simulink model "Battery_Simulator"  (R2014a)
settings: Solver=FixedStepDiscrete  StartTime=0.0  StopTime=10.0  RelTol=1e-3
PreLoadFcn:
  | try, eval([bdroot '_setup']); catch, eval('model_setup', ''); end
InitFcn:
  | try, eval([bdroot '_setup']); catch, eval('model_setup', ''); end
undefined symbols (not defined in the file or in its folder): ECU565, motohawk_build_version, motohawk_trunc_name, motohawk_vardec_path
undefined symbols (not defined in the file): motohawk_get_target_image, motohawk_target_type
libraries: MotoHawk_lib x42, motohawk_annotations_lib x36
(part 1 of 2)
CloseFcn:
  | try, eval([bdroot '_close']); catch, eval('model_close', ''); end
Description:
  | Battery_Simulator
settings Model: MotoHawkBuildVersion=000  MotoHawkBuildStats=struct('TotalFLASH',{0},'TotalEEPROM',{0},'TotalRAM',{0},'AppFLASH',{0},'AppEEPROM',{0},'AppRAM',{0},'HeapRAM',{0},'BuildSuccessCount',{0},'BuildErrorCount',{0})  MotoHawkModelSavedName=Battery_Simulator  MotoHawkModelGUID=A0987AB7-E185-4605-B89A-B215F82E656D  MotoHawkModelOpenTime=2016 9 1 13 11 10.754  MotoHawkModelElapsedTime=6085.987  MotoHawkBuildInfo=struct('model_name',{'motohawk_template_model'},'motohawk_version',{'0.8.4_beta1'},'motohawk_component_version',{'0.0.3'},'matlab_version',{'6.5.1'},'build_version',{'000'},'layout_type',{'DEV'},'eri_table0_rev',{9},'max_eri_table_size',{255},'fptype',{0},'fgnd_base_period_ms',{5},'bgnd_base_period_ms',{50},'module_type',{'ECU555-80'},'processor_family',{'PPC'},'processor_type',{'MPC555'},'toolchain',{'GHS3.6'},'component',{0},'resource_file',{'PCM555Resources.h'},'archive_file',{'PCM.a'},'enable_build',{1},'flash_size',{458752},'ee_size',{8192},'ram_size',{26624},'decram_size',{0},'module_memory_def',{'MPC555_ModMemoryDef_Dev'},'use_debug_vardecs',{1},'root_build_dir',{'C:\MotoTron\MOTOHA~3\Blocks\Project'},'build_dir',{'C:\MotoTron\MOTOHA~3\Blocks\Project\motohawk_template_model_Build'},'dll_name',{'motohawk__000'},'srz_name',{'motohawk_template_model_000'},'fgnd_stack_size',{3072},'fgnd_angle_stack_size',{0},'bgnd_stack_size',{2048},'idle_stack_size',{1024},'irq_stack_size',{1536},'heap_size',{4096},'install_dll_dir',{'C:\ECUFiles\TDBDLL\'},'install_srz_dir',{'C:\ECUFiles\Programs\'},'motodevelopment_dir',{'C:\PROGRA~1\MotoTron\DEVELO~1\'},'motohawk_dir',{'C:\MotoTron\MOTOHA~3'},'ghs_dir',{'C:\GHS\ppc36'},'cw_dir',{'C:\Program Files\Freescale\CW for HC12 V4.5'},'matlab_root',{'C:\MATLAB6p5p1'},'model_guid',{'a528c725-4135-4734-9f-2c-07-29-37-5b-38'},'build_guid',{[]},'token_guid',{'6198A7A8FF044D4685C525ADFA06DAD5'})  Creator=cspenc  LastModifiedBy=ab9547
settings ConfigSet: Description="This Simulink Configuration Set is preconfigured  for the MotoHawk target \"ECU565-128\"."
settings OptimizationCC: InlineParams=on  InlineInvariantSignals=on  EnhancedBackFolding=on  ExpressionDepthLimit=2147483647  InitFltsAndDblsToZero=on  NoFixptDivByZeroProtection=on  EfficientFloat2IntCast=on  OptimizeModelRefInitCode=on  LifeSpan=1
settings DebuggingCC: UnderspecifiedInitializationDetection=Classic  SolverPrmCheckMsg=none  InheritedTsInSrcMsg=none  TasksWithSamePriorityMsg=none  FcnCallInpInsideContextMsg=EnableAllAsWarning  StateNameClashWarn=warning
settings HardwareCC: ProdLargestAtomicInteger=Integer  ProdLargestAtomicFloat=Float  ProdEndianess=BigEndian  ProdHWDeviceType=Specified
settings ModelReferenceCC: UpdateModelReferenceTargets=AssumeUpToDate  CheckModelReferenceTargetMessage=none  ModelReferenceNumInstancesAllowed=Zero
settings RTWCC: SystemTargetFile=motohawk_ert_rtw.tlc  MakeCommand=motohawk_make_rtw  TemplateMakefile=motohawk_ert_rtw.tmf  Description=MotoHawk(tm) Rapid Prototyping  ProcessScript=motohawk_ert_rtw_make_rtw_hook
settings CodeAppCC: IgnoreCustomStorageClasses=off  MaxIdLength=100  CustomSymbolStrType=$N$R$M  CustomSymbolStrField=$H$N$M  InternalIdentifier=Classic
settings STFCustomTargetCC: ERTMultiwordTypeDef=User defined  ERTMultiwordLength=0  ModelReferenceCompliant=off  ConcurrentExecutionCompliant=off  IncludeMdlTerminateFcn=off  CombineOutputUpdateFcns=on  SuppressErrorStatus=on  ERTCustomFileBanners=on  SupportContinuousTime=off  SupportNonInlinedSFcns=off  MATLABClassNameForMDSCustomization=Simulink.SoftwareTarget.ERTCustomization  GRTInterface=off  SystemTargetFile=motohawk_ert_rtw.tlc
settings ERTTargetCC: ERTMultiwordTypeDef=User defined  ERTMultiwordLength=0  GenerateSampleERTMain=off  ModelReferenceCompliant=off  IncludeMdlTerminateFcn=off  GeneratePreprocessorConditionals=Disable all  SuppressErrorStatus=on  ERTCustomFileTemplate=example_file_process.tlc

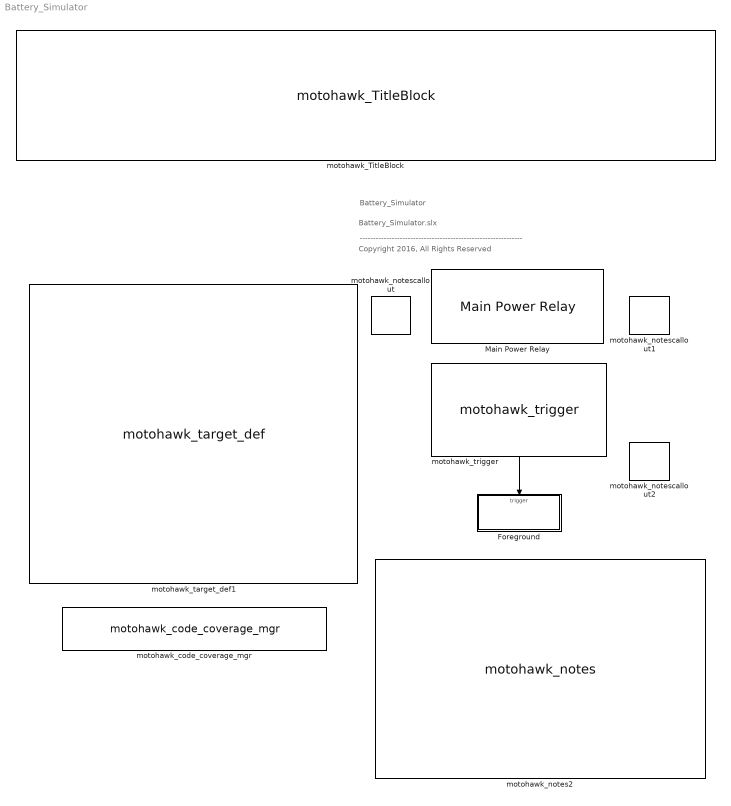
== system Battery_Simulator ==
  note: Battery_Simulator
  note: Battery_Simulator.slx
  note: -------------------------------------------------------------
  note: Copyright 2016, All Rights Reserved
  Foreground : Subsystem  TreatAsAtomicUnit=on
      mask init:
      | SampleTime = 0.005;
      | lbl = sprintf('%d ms', SampleTime * 1000);
      settings: RTWSystemCode=Nonreusable function  RTWFcnNameOpts=Use subsystem name  RTWFileNameOpts=Use function name
      mask Display: disp(lbl);
  Main Power Relay : MotoHawk_lib/Extra Development Blocks/Main Power Relay  on_delay_count=2  off_delay_count=5  ecup_threshold=100  group='System | Main Power Relay'
  motohawk_TitleBlock : motohawk_annotations_lib/motohawk_TitleBlock  BlockType_='Mototron_Title_Block'  ttl="[        strrep(get_param(bdroot, 'Description') , '_', '\\_')  '\\newline\\rm'        'Top-level root of model:  '   strrep(bdroot, '_', '\\_') '.mdl'        ]"  copyright="'THE INFORMATION CONTAINED IN THIS\\newlineDRAWING IS THE SOLE PROPERTY OF\\newlineWOODWARD.  ANY REPRODUCTION IN\\newline PART OR AS A WHOLE WITHOUT THE\\newlineWRITTEN PERMISSION OF WOODWARD\\newline IS PROHIBITED.\\fontsize{16}\\rm\\copyright\\rm\\fontsize{10} 2009'"  address='\fontsize{22}\it\fontname{Arial Black}Woodward \fontname{Arial}\fontsize{10}\newline1000 East Drake Road, Fort Collins, CO, 80525\newlinemcs.woodward.com (866) 588-0494'  image_file='mh.jpg'  pretty_print=on  edit_text="[strrep(get_param(bdroot, 'Description') , '_', '\\_')  '\\newline\\rm''Top-level root of model:  '   strrep(bdroot, '_', '\\_') '.mdl']"  edit_as=5
  motohawk_code_coverage_mgr : MotoHawk_lib/Extra Development Blocks/motohawk_code_coverage_mgr  codegen=Always Generate Code Coverage Code  group='System | Code Coverage'
  motohawk_notes2 : motohawk_annotations_lib/motohawk_notes  BlockType_='Mototron_Notes'  desc="'\\fontname{wingdings 2}u\\fontname{arial}  The existence of a Target Definition block\\newlinesomewhere in the model sets it up as a\\newlineMotoHawk project, capable of being built to a\\newlineMotoHawk capable target module.\\newline\\newline\\fontname{wingdings 2}v\\fontname{arial}  The Main Power Relay block monitors the\\newlinemodule power and controls the Main Power Relay\\newlineIt also performs startup and shutdown procedures\\newlinenecessary for EEPROM storage.  Most designs\\newlineshould contain this block\\newline\\newline\\fontname{wingdings 2}w\\fontname{arial}  All actions must be performed inside of a\\newlinefunction-call subsystem, triggered by a MotoHawk\\newlineentry-point trigger block, in order to be included in the\\newlinegenerated code.'"  edit_text="\\fontname{wingdings 2}u\\fontname{arial}  The existence of a Target Definition blocksomewhere in the model sets it up as aMotoHawk project, capable of being built to aMotoHawk capable target module.\\fontname{wingdings 2}v\\fontname{arial}  The Main Power Relay block monitors themodule power and controls the Main Power RelayIt also performs startup and shutdown proceduresnecessary for EEPROM storage.  Most designsshould contain this block\\fontname{wingdings 2}w\\fontname{arial}  All actions must be performed inside of afunction-call subsystem, triggered by a MotoHawkentry-point trigger block, in order to be included in thegenerated code."  edit_as=2
  motohawk_notescallout : motohawk_annotations_lib/motohawk_notescallout  BlockType_='Mototron_NoteCall'  desc='\bf1'
  motohawk_notescallout1 : motohawk_annotations_lib/motohawk_notescallout  BlockType_='Mototron_NoteCall'  desc='\bf2'
  motohawk_notescallout2 : motohawk_annotations_lib/motohawk_notescallout  BlockType_='Mototron_NoteCall'  desc='\bf3'
  motohawk_target_def1 : MotoHawk_lib/motohawk_target_def  Priority=-65535  target=ECU565-128  layout=DEV  fptype=single (32 bits)  fgnd_stack_size=3*1024  fgnd_angle_stack_size=0  bgnd_stack_size=2*1024  idle_stack_size=1024  irq_stack_size=1536  app_int_stack_size=1024  shutdown_stack_size=1024  heap_size=4*1024  show_margins=off  fgnd_stack_margin=(3*1024) * 0.1  fgnd_angle_stack_margin=0  bgnd_stack_margin=(2*1024) * 0.1  idle_stack_margin=(1024) * 0.1  irq_stack_margin=(1536) * 0.1  app_int_stack_margin=(1024) * 0.1  shutdown_stack_margin=(1024) * 0.1  heap_margin=(4*1024) * 0.1  comp_name=bdroot  comp_img='KVASER_CAN_USB.jpg'  comp_security=No Encryption  comp_build_pass='mhbuild'  comp_sim_pass='mhsim'  comp_multi=off  show_filenames=off  dll_name=motohawk_trunc_name(bdroot, ['_' motohawk_build_version], 50)  srz_name=motohawk_trunc_name(bdroot, ['_' motohawk_build_version], 50)  build_dir='.'  comp_dir='.'
  motohawk_trigger : MotoHawk_lib/Trigger Blocks/motohawk_trigger  Tag=Trigger  Priority=0  trig_name=[]  trigger=FGND_RTI_PERIODIC  priority_order=0  inherited=off  run_disabled=off  override_app_monitor=off  target=ECU565_128
  wires:
  motohawk_trigger/1 -> Foreground/Trigger

== system Battery_Simulator/Foreground ==
  f : TriggerPort  TriggerType=function-call
  Controller : Subsystem  mask(Display Image File){image_file=motohawk_get_target_image(motohawk_target_type(bdroot))}
      mask prompts: image_file "Image File"
      mask help:
      | Enter an image file on the current MATLAB path to display on this block.
      |
      | Double-clicking this block opens the contents of the subsystem.  Right-click and select 'Mask parameters...' to select a new image file.
      |
      | To use just the mask of this block in a model, but supply your own contents, break the link to the library.
      mask init:
      | try,
      | 	img = imread(image_file);
      | 	motohawk_block_image(gcb, image_file);
      | catch,
      | 	img = imread('image_not_found.jpg');
      | end
      settings: OpenFcn=open_system(gcb,'force')  MoveFcn=motohawk_block_image(gcb, motohawk_get_param_ws(gcb, 'image_file'));
      mask Display: image(img);
  Plant : Subsystem  mask(Display Image File){image_file='engine.jpg'}
      mask prompts: image_file "Image File"
      mask help:
      | Enter an image file on the current MATLAB path to display on this block.
      |
      | Double-clicking this block opens the contents of the subsystem.  Right-click and select 'Mask parameters...' to select a new image file.
      |
      | To use just the mask of this block in a model, but supply your own contents, break the link to the library.
      mask init:
      | try,
      | 	img = imread(image_file);
      | 	motohawk_block_image(gcb, image_file);
      | catch,
      | 	img = imread('image_not_found.jpg');
      | end
      settings: OpenFcn=open_system(gcb,'force')  MoveFcn=motohawk_block_image(gcb, motohawk_get_param_ws(gcb, 'image_file'));
      mask Display: image(img);
  motohawk_TitleBlock : motohawk_annotations_lib/motohawk_TitleBlock  BlockType_='Mototron_Title_Block'  ttl=[strrep(get_param(bdroot, 'Description') , '_', '\_') '\newline\rm' get_param(gcs, 'Name')]  copyright="'THE INFORMATION CONTAINED IN THIS\\newlineDRAWING IS THE SOLE PROPERTY OF\\newlineWOODWARD.  ANY REPRODUCTION IN\\newline PART OR AS A WHOLE WITHOUT THE\\newlineWRITTEN PERMISSION OF WOODWARD\\newline IS PROHIBITED.\\fontsize{16}\\rm\\copyright\\rm\\fontsize{10} 2009'"  address='\fontsize{22}\it\fontname{Arial Black}Woodward \fontname{Arial}\fontsize{10}\newline1000 East Drake Road, Fort Collins, CO, 80525\newlinemcs.woodward.com (866) 588-0494'  image_file='mh.jpg'  pretty_print=on  edit_text=[strrep(get_param(bdroot, 'Description') , '_', '\_') '\newline\rm' get_param(gcs, 'Name')]  edit_as=5
  motohawk_code_coverage : MotoHawk_lib/Extra Development Blocks/motohawk_code_coverage
  wires:
  Plant/1(SensorBus) -> Controller/1(Sensors)
  Controller/1(Actuators) -> Plant/1(ActuatorBus)

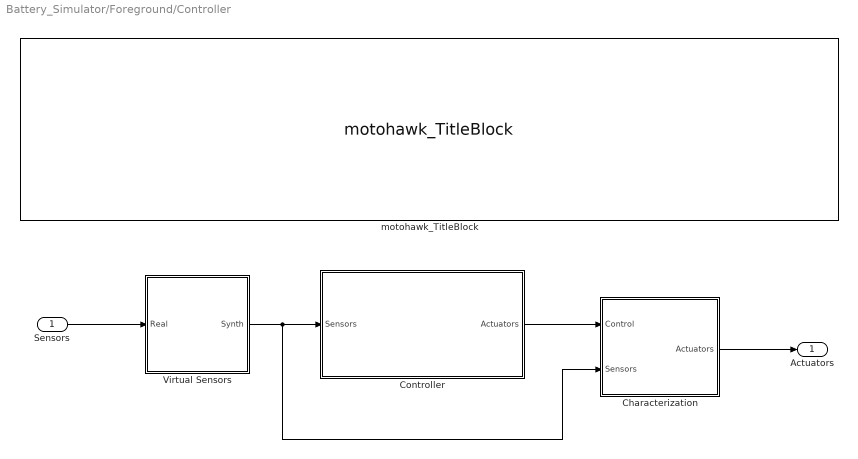
== system Battery_Simulator/Foreground/Controller ==
  Sensors : Inport
  Characterization : Subsystem
  Controller : Subsystem
  Virtual Sensors : Subsystem
  motohawk_TitleBlock : motohawk_annotations_lib/motohawk_TitleBlock  BlockType_='Mototron_Title_Block'  ttl=[get_param(bdroot, 'Description') '\rm\newlineTop-level design of Controller\newlineVirtual Sensors model signals that are not available as H/W sensors\newlineCharacterization converts or linearizes Controller units to actuator units\newline']  copyright="'THE INFORMATION CONTAINED IN THIS\\newlineDRAWING IS THE SOLE PROPERTY OF\\newlineWOODWARD.  ANY REPRODUCTION IN\\newline PART OR AS A WHOLE WITHOUT THE\\newlineWRITTEN PERMISSION OF WOODWARD\\newline IS PROHIBITED.\\fontsize{16}\\rm\\copyright\\rm\\fontsize{10} 2009'"  address='\fontsize{22}\it\fontname{Arial Black}Woodward \fontname{Arial}\fontsize{10}\newline1000 East Drake Road, Fort Collins, CO, 80525\newlinemcs.woodward.com (866) 588-0494'  image_file='mh.jpg'  pretty_print=on  edit_text=|  edit_as=6
      | [get_param(bdroot, 'Description') '\rm
      | 
      | 
      | Top-level design of Controller
      | 
      | 
      | Virtual Sensors model signals that are not available as H/W sensors
      | 
      | 
      | Characterization converts or linearizes Controller units to actuator units
      | 
      | 
      | ']
  Actuators : Outport
  wires:
  Controller/1(Actuators) -> Characterization/1(Control)
  Virtual Sensors/1(Synth) -> Controller/1(Sensors), Characterization/2(Sensors)
  Sensors/1 -> Virtual Sensors/1(Real)
  Characterization/1(Actuators) -> Actuators/1

== system Battery_Simulator/Foreground/Plant ==
  ActuatorBus : Inport
  Actuators : Subsystem
  Sensors : Subsystem
  motohawk_TitleBlock : motohawk_annotations_lib/motohawk_TitleBlock  BlockType_='Mototron_Title_Block'  ttl=[get_param(bdroot, 'Description') '\rm\newlineRead H/W sensors and Drive H/W actuators\newlineThe Sensors and Actuators busses should contain signals in engineering units\newline']  copyright="'THE INFORMATION CONTAINED IN THIS\\newlineDRAWING IS THE SOLE PROPERTY OF\\newlineWOODWARD.  ANY REPRODUCTION IN\\newline PART OR AS A WHOLE WITHOUT THE\\newlineWRITTEN PERMISSION OF WOODWARD\\newline IS PROHIBITED.\\fontsize{16}\\rm\\copyright\\rm\\fontsize{10} 2009'"  address='\fontsize{22}\it\fontname{Arial Black}Woodward \fontname{Arial}\fontsize{10}\newline1000 East Drake Road, Fort Collins, CO, 80525\newlinemcs.woodward.com (866) 588-0494'  image_file='mh.jpg'  pretty_print=on  edit_text=|  edit_as=6
      | [get_param(bdroot, 'Description') '\rm
      | 
      | 
      | Read H/W sensors and Drive H/W actuators
      | 
      | 
      | The Sensors and Actuators busses should contain signals in engineering units
      | 
      | 
      | ']
  SensorBus : Outport
  wires:
  Sensors/1(Sensors) -> SensorBus/1
  ActuatorBus/1 -> Actuators/1(Actuators)

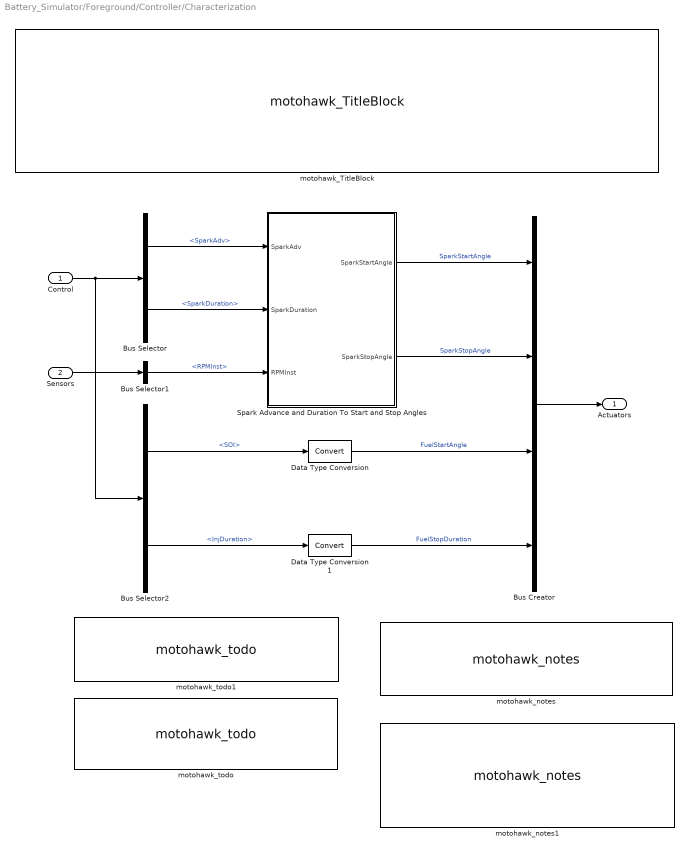
== system Battery_Simulator/Foreground/Controller/Characterization ==
  Control : Inport
  Sensors : Inport  Port=2
  Bus Creator : BusCreator
  Bus Selector : BusSelector  OutputSignals=SparkAdv,SparkDuration
  Bus Selector1 : BusSelector  OutputSignals=RPMInst
  Bus Selector2 : BusSelector  OutputSignals=SOI,InjDuration
  Data Type Conversion : DataTypeConversion  SaturateOnIntegerOverflow=on  RndMeth=Zero
  Data Type Conversion1 : DataTypeConversion  SaturateOnIntegerOverflow=on  RndMeth=Zero
  Spark Advance and Duration To Start and Stop Angles : Subsystem
  motohawk_TitleBlock : motohawk_annotations_lib/motohawk_TitleBlock  BlockType_='Mototron_Title_Block'  ttl=[get_param(bdroot, 'Description') '\rm\newlineActuator Characterization\newlineConverts or linearizes controller units to actuator units\newline']  copyright="'THE INFORMATION CONTAINED IN THIS\\newlineDRAWING IS THE SOLE PROPERTY OF\\newlineWOODWARD.  ANY REPRODUCTION IN\\newline PART OR AS A WHOLE WITHOUT THE\\newlineWRITTEN PERMISSION OF WOODWARD\\newline IS PROHIBITED.\\fontsize{16}\\rm\\copyright\\rm\\fontsize{10} 2009'"  address='\fontsize{22}\it\fontname{Arial Black}Woodward \fontname{Arial}\fontsize{10}\newline1000 East Drake Road, Fort Collins, CO, 80525\newlinemcs.woodward.com (866) 588-0494'  image_file='mh.jpg'  pretty_print=on  edit_text=|  edit_as=6
      | [get_param(bdroot, 'Description') '\rm
      | 
      | 
      | Actuator Characterization
      | 
      | 
      | Converts or linearizes controller units to actuator units
      | 
      | 
      | ']
  motohawk_notes : motohawk_annotations_lib/motohawk_notes  BlockType_='Mototron_Notes'  desc='- Outputs from here are still entirely in engineering\newlineunits, but are converted from a form used by the\newlinecontroller to one required by the physical actuators'  edit_text=|  edit_as=0
      | - Outputs from here are still entirely in engineering
      | 
      | 
      | units, but are converted from a form used by the
      | 
      | 
      | controller to one required by the physical actuators
  motohawk_notes1 : motohawk_annotations_lib/motohawk_notes  BlockType_='Mototron_Notes'  desc='- This is a good place to put a PID controller that\newlineis always enabled, such as an electronic throttle\newlinecontroller (ETC)\newline\newline- The controller outputs a desired setpoint,\newlinea block in this subsystem performs the\newlineclosed-loop control to that position.'  edit_text=|  edit_as=0
      | - This is a good place to put a PID controller that
      | 
      | 
      | is always enabled, such as an electronic throttle
      | 
      | 
      | controller (ETC)
      | 
      | 
      | 
      | 
      | 
      | - The controller outputs a desired setpoint,
      | 
      | 
      | a block in this subsystem performs the
      | 
      | 
      | closed-loop control to that position.
  motohawk_todo : motohawk_annotations_lib/motohawk_todo  BlockType_='Mototron_ToDo'  desc='\fontsize{16}\bfTo Do:\newlineConvert from desired controller units\newlineto those required by each actuator.'  edit_text=|  edit_as=2
      | \fontsize{16}\bfTo Do:
      | 
      | 
      | Convert from desired controller units
      | 
      | 
      | to those required by each actuator.
  motohawk_todo1 : motohawk_annotations_lib/motohawk_todo  BlockType_='Mototron_ToDo'  desc='\fontsize{16}\bfTo Do:\newlinePass-through actuators\newlinethat do not require modification.'  edit_text=|  edit_as=2
      | \fontsize{16}\bfTo Do:
      | 
      | 
      | Pass-through actuators
      | 
      | 
      | that do not require modification.
  Actuators : Outport
  wires:
  Spark Advance and Duration To Start and Stop Angles/1(SparkStartAngle) -> Bus Creator/1  "SparkStartAngle"
  Bus Creator/1 -> Actuators/1
  Spark Advance and Duration To Start and Stop Angles/2(SparkStopAngle) -> Bus Creator/2  "SparkStopAngle"
  Bus Selector2/1 -> Data Type Conversion/1  "<SOI>"
  Bus Selector2/2 -> Data Type Conversion1/1  "<InjDuration>"
  Sensors/1 -> Bus Selector1/1
  Bus Selector1/1 -> Spark Advance and Duration To Start and Stop Angles/3(RPMInst)  "<RPMInst>"
  Bus Selector/1 -> Spark Advance and Duration To Start and Stop Angles/1(SparkAdv)  "<SparkAdv>"
  Bus Selector/2 -> Spark Advance and Duration To Start and Stop Angles/2(SparkDuration)  "<SparkDuration>"
  Control/1 -> Bus Selector/1, Bus Selector2/1
  Data Type Conversion/1 -> Bus Creator/3  "FuelStartAngle"
  Data Type Conversion1/1 -> Bus Creator/4  "FuelStopDuration"

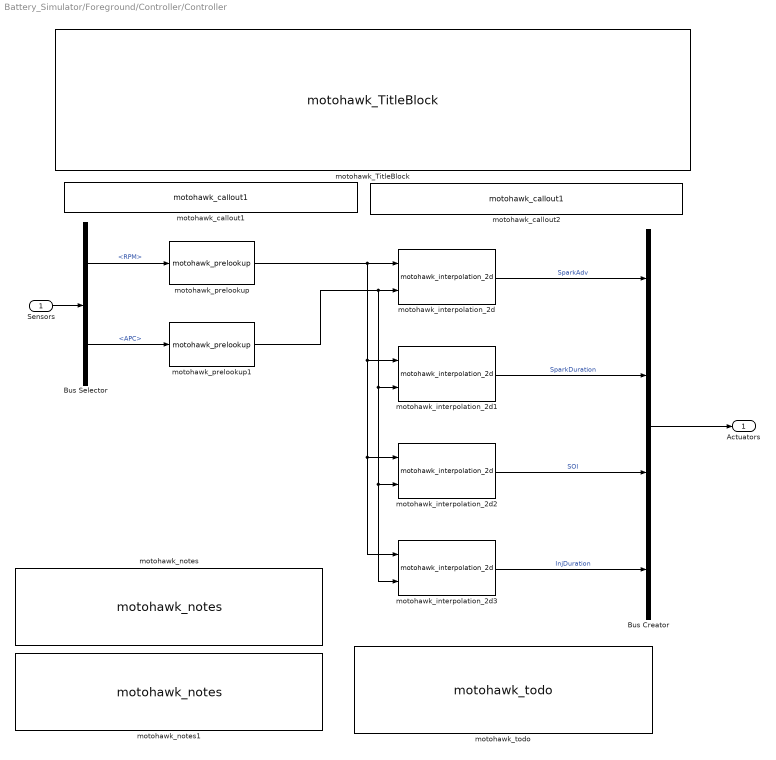
== system Battery_Simulator/Foreground/Controller/Controller ==
  Sensors : Inport
  Bus Creator : BusCreator
  Bus Selector : BusSelector  OutputSignals=RPM,APC
  motohawk_TitleBlock : motohawk_annotations_lib/motohawk_TitleBlock  BlockType_='Mototron_Title_Block'  ttl=[get_param(bdroot, 'Description') '\rm\newlineEngine control system\newlineConsists of simple tables for spark and fuel\newline']  copyright="'THE INFORMATION CONTAINED IN THIS\\newlineDRAWING IS THE SOLE PROPERTY OF\\newlineWOODWARD.  ANY REPRODUCTION IN\\newline PART OR AS A WHOLE WITHOUT THE\\newlineWRITTEN PERMISSION OF WOODWARD\\newline IS PROHIBITED.\\fontsize{16}\\rm\\copyright\\rm\\fontsize{10} 2009'"  address='\fontsize{22}\it\fontname{Arial Black}Woodward \fontname{Arial}\fontsize{10}\newline1000 East Drake Road, Fort Collins, CO, 80525\newlinemcs.woodward.com (866) 588-0494'  image_file='mh.jpg'  pretty_print=on  edit_text=|  edit_as=6
      | [get_param(bdroot, 'Description') '\rm
      | 
      | 
      | Engine control system
      | 
      | 
      | Consists of simple tables for spark and fuel
      | 
      | 
      | ']
  motohawk_callout1 : motohawk_annotations_lib/motohawk_callout1  BlockType_='Mototron_harea'  desc='Prelookups for each axis of the tables'  edit_text=Prelookups for each axis of the tables  edit_as=0
  motohawk_callout2 : motohawk_annotations_lib/motohawk_callout1  BlockType_='Mototron_harea'  desc='2-D interpolated tables for each actuator'  edit_text=2-D interpolated tables for each actuator  edit_as=0
  motohawk_interpolation_2d : MotoHawk_lib/Lookup Tables/motohawk_interpolation_2d  nam='SparkAdv'  table_data=zeros(11,11)  show_more=off  data_type=Inherit from 'Table Data'  storage=NonAdaptive  read_level=1  write_level=1  ovr_cals=on  use_help=off  help=''  units=''  use_min_max=off  min_val=-inf  max_val=inf  use_precision=off  precision=''  gain=1  offset=0  exp=1  use_links=off  row_prelookup_block=''  col_prelookup_block=''  output_name=''  use_mototune_group=off  mototune_group=motohawk_vardec_path(gcb)  data_stores=motohawk_sfun_interpolation_2d_data_stores
  motohawk_interpolation_2d1 : MotoHawk_lib/Lookup Tables/motohawk_interpolation_2d  nam='SparkDuration'  table_data=ones(11,11)  show_more=off  data_type=Inherit from 'Table Data'  storage=NonAdaptive  read_level=1  write_level=1  ovr_cals=on  use_help=off  help=''  units=''  use_min_max=off  min_val=-inf  max_val=inf  use_precision=off  precision=''  gain=1  offset=0  exp=1  use_links=off  row_prelookup_block=''  col_prelookup_block=''  output_name=''  use_mototune_group=off  mototune_group=motohawk_vardec_path(gcb)  data_stores=motohawk_sfun_interpolation_2d_data_stores
  motohawk_interpolation_2d2 : MotoHawk_lib/Lookup Tables/motohawk_interpolation_2d  nam='SOI'  table_data=zeros(11,11)  show_more=off  data_type=Inherit from 'Table Data'  storage=NonAdaptive  read_level=1  write_level=1  ovr_cals=on  use_help=off  help=''  units=''  use_min_max=off  min_val=-inf  max_val=inf  use_precision=off  precision=''  gain=1  offset=0  exp=1  use_links=off  row_prelookup_block=''  col_prelookup_block=''  output_name=''  use_mototune_group=off  mototune_group=motohawk_vardec_path(gcb)  data_stores=motohawk_sfun_interpolation_2d_data_stores
  motohawk_interpolation_2d3 : MotoHawk_lib/Lookup Tables/motohawk_interpolation_2d  nam='InjDuration'  table_data=5*ones(11,11)  show_more=off  data_type=Inherit from 'Table Data'  storage=NonAdaptive  read_level=1  write_level=1  ovr_cals=on  use_help=off  help=''  units=''  use_min_max=off  min_val=-inf  max_val=inf  use_precision=off  precision=''  gain=1  offset=0  exp=1  use_links=off  row_prelookup_block=''  col_prelookup_block=''  output_name=''  use_mototune_group=off  mototune_group=motohawk_vardec_path(gcb)  data_stores=motohawk_sfun_interpolation_2d_data_stores
  motohawk_notes : motohawk_annotations_lib/motohawk_notes  BlockType_='Mototron_Notes'  desc='Simplify as much as possible, by offloading work to the\newlineVirtual Sensors and Actuator Characterization subsystems'  edit_text=|  edit_as=0
      | Simplify as much as possible, by offloading work to the
      | 
      | 
      | Virtual Sensors and Actuator Characterization subsystems
  motohawk_notes1 : motohawk_annotations_lib/motohawk_notes  BlockType_='Mototron_Notes'  desc='If the controller contains multiple states,\newlinecreate a StateFlow representation of the state machine here.'  edit_text=|  edit_as=0
      | If the controller contains multiple states,
      | 
      | 
      | create a StateFlow representation of the state machine here.
  motohawk_prelookup : MotoHawk_lib/Lookup Tables/motohawk_prelookup  nam='RPM'  breakpoint_data=[0:500:5000]  show_more=on  data_type=Inherit from 'Table Data'  storage=Constant  read_level=1  write_level=1  ovr_cals=on  use_help=off  help=''  units=''  use_min_max=off  min_val=-inf  max_val=inf  use_precision=off  precision=''  gain=1  offset=0  exp=1  use_links=on  input_name='RPM'  use_mototune_group=off  mototune_group=motohawk_vardec_path(gcb)  data_stores=motohawk_sfun_prelookup_data_stores
  motohawk_prelookup1 : MotoHawk_lib/Lookup Tables/motohawk_prelookup  nam='APC'  breakpoint_data=[0:0.5:5]  show_more=on  data_type=Inherit from 'Table Data'  storage=Constant  read_level=1  write_level=1  ovr_cals=on  use_help=off  help=''  units=''  use_min_max=off  min_val=-inf  max_val=inf  use_precision=off  precision=''  gain=1  offset=0  exp=1  use_links=on  input_name='APC'  use_mototune_group=off  mototune_group=motohawk_vardec_path(gcb)  data_stores=motohawk_sfun_prelookup_data_stores
  motohawk_todo : motohawk_annotations_lib/motohawk_todo  BlockType_='Mototron_ToDo'  desc='\fontsize{16}\bfTo Do:\newlinePerform the actions required by the controller.'  edit_text=|  edit_as=2
      | \fontsize{16}\bfTo Do:
      | 
      | 
      | Perform the actions required by the controller.
  Actuators : Outport
  wires:
  Bus Creator/1 -> Actuators/1
  motohawk_interpolation_2d/1 -> Bus Creator/1  "SparkAdv"
  motohawk_interpolation_2d1/1 -> Bus Creator/2  "SparkDuration"
  motohawk_interpolation_2d2/1 -> Bus Creator/3  "SOI"
  motohawk_interpolation_2d3/1 -> Bus Creator/4  "InjDuration"
  Sensors/1 -> Bus Selector/1
  Bus Selector/1 -> motohawk_prelookup/1  "<RPM>"
  Bus Selector/2 -> motohawk_prelookup1/1  "<APC>"
  motohawk_prelookup/1 -> motohawk_interpolation_2d/1, motohawk_interpolation_2d1/1, motohawk_interpolation_2d2/1, motohawk_interpolation_2d3/1
  motohawk_prelookup1/1 -> motohawk_interpolation_2d/2, motohawk_interpolation_2d1/2, motohawk_interpolation_2d2/2, motohawk_interpolation_2d3/2

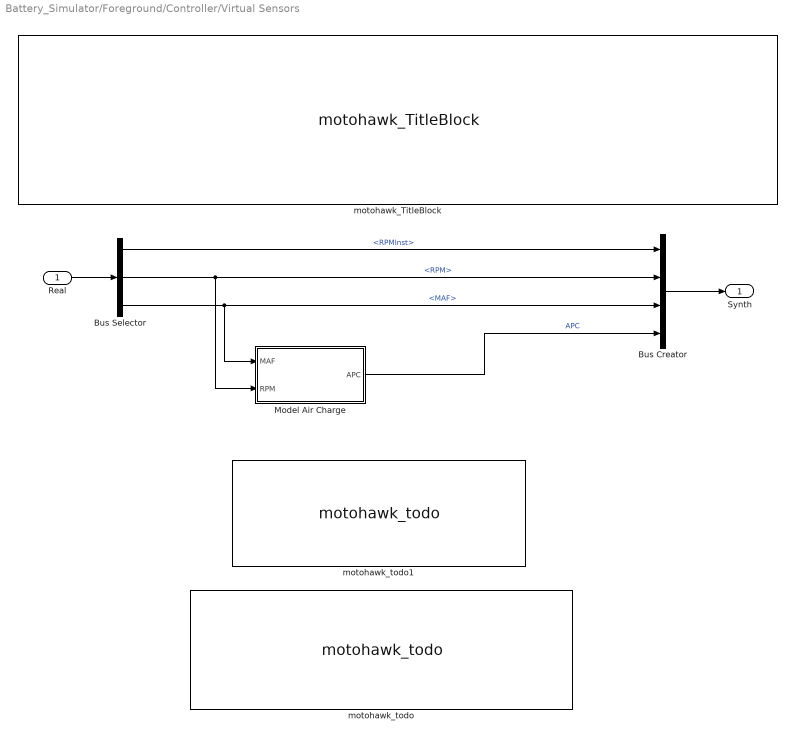
== system Battery_Simulator/Foreground/Controller/Virtual Sensors ==
  Real : Inport
  Bus Creator : BusCreator
  Bus Selector : BusSelector  OutputSignals=RPMInst,RPM,MAF
  Model Air Charge : Subsystem
  motohawk_TitleBlock : motohawk_annotations_lib/motohawk_TitleBlock  BlockType_='Mototron_Title_Block'  ttl=[get_param(bdroot, 'Description') '\newline\rmVirtual Sensors\newlineModel signals that are not available as H/W sensors,\newlinebut that would be used by the controller if they were physically available']  copyright="'THE INFORMATION CONTAINED IN THIS\\newlineDRAWING IS THE SOLE PROPERTY OF\\newlineWOODWARD.  ANY REPRODUCTION IN\\newline PART OR AS A WHOLE WITHOUT THE\\newlineWRITTEN PERMISSION OF WOODWARD\\newline IS PROHIBITED.\\fontsize{16}\\rm\\copyright\\rm\\fontsize{10} 2009'"  address='\fontsize{22}\it\fontname{Arial Black}Woodward \fontname{Arial}\fontsize{10}\newline1000 East Drake Road, Fort Collins, CO, 80525\newlinemcs.woodward.com (866) 588-0494'  image_file='mh.jpg'  pretty_print=on  edit_text="strrep([get_param(bdroot, 'Description')  '\\rm\\newline'  get_param(gcs, 'Name')], '_', '\\_')"  edit_as=255
  motohawk_todo : motohawk_annotations_lib/motohawk_todo  BlockType_='Mototron_ToDo'  desc="'\\fontsize{16}\\bfTo Do:\\newlineModel Extra \"Virtual\" Sensors\\newlineso that the downstream controller can\\newlineuse modeled variables as sensor values'"  edit_text=|  edit_as=2
      | \fontsize{16}\bfTo Do:
      | 
      | 
      | Model Extra "Virtual" Sensors
      | 
      | 
      | so that the downstream controller can
      | 
      | 
      | use modeled variables as sensor values
  motohawk_todo1 : motohawk_annotations_lib/motohawk_todo  BlockType_='Mototron_ToDo'  desc='\fontsize{16}\bfTo Do:\newlinePass-through sensors\newlinethat do not require modification.'  edit_text=|  edit_as=2
      | \fontsize{16}\bfTo Do:
      | 
      | 
      | Pass-through sensors
      | 
      | 
      | that do not require modification.
  Synth : Outport
  wires:
  Real/1 -> Bus Selector/1
  Bus Selector/1 -> Bus Creator/1  "<RPMInst>"
  Bus Selector/2 -> Bus Creator/2, Model Air Charge/2(RPM)  "<RPM>"
  Bus Selector/3 -> Bus Creator/3, Model Air Charge/1(MAF)  "<MAF>"
  Model Air Charge/1(APC) -> Bus Creator/4  "APC"
  Bus Creator/1 -> Synth/1

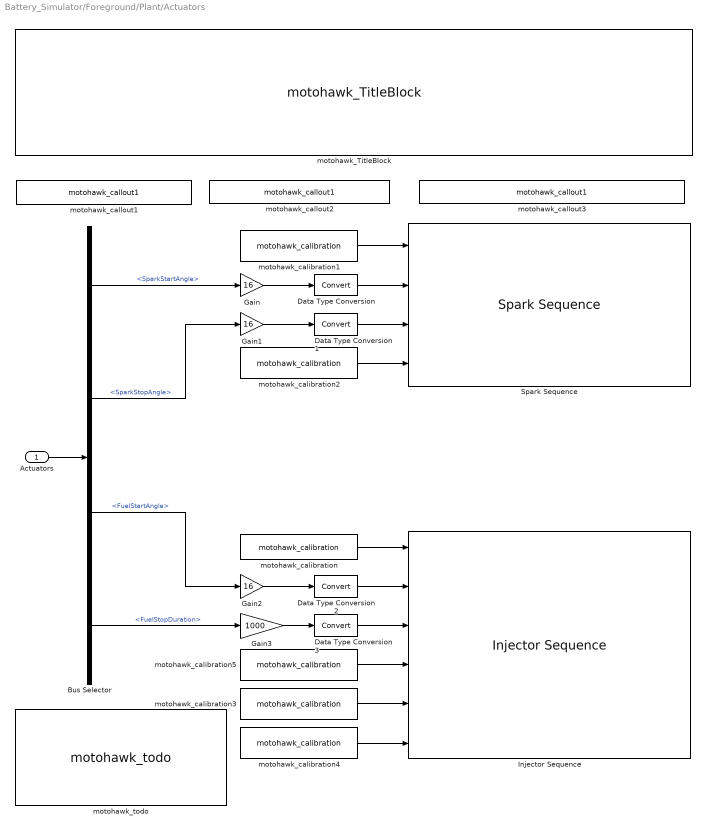
== system Battery_Simulator/Foreground/Plant/Actuators ==
  Actuators : Inport
  Bus Selector : BusSelector  OutputSignals=SparkStartAngle,SparkStopAngle,FuelStartAngle,FuelStopDuration
  Data Type Conversion{,1..3} (4 alike) : DataTypeConversion  SaturateOnIntegerOverflow=on  RndMeth=Zero
  Gain : Gain  Gain=16  SaturateOnIntegerOverflow=on  OutDataTypeStr=Inherit: Same as input  ParamDataTypeStr=Inherit: Same as input
  Gain1 : Gain  Gain=16  SaturateOnIntegerOverflow=on  OutDataTypeStr=Inherit: Same as input  ParamDataTypeStr=Inherit: Same as input
  Gain2 : Gain  Gain=16  SaturateOnIntegerOverflow=on  OutDataTypeStr=Inherit: Same as input  ParamDataTypeStr=Inherit: Same as input
  Gain3 : Gain  Gain=1000  SaturateOnIntegerOverflow=on  OutDataTypeStr=Inherit: Same as input  ParamDataTypeStr=Inherit: Same as input
  Injector Sequence : MotoHawk_lib/Advanced Digital I//O/Injector Sequence  text_resource=FINJ1  code_resource=NONE  val_resource=-1  target=ECU565-128  resource_enum_str=(None)=-1,FINJ1=12,FINJ2=13,FINJ3=14,FINJ4=15,FINJ5=16,FINJ6=17,FINJ7=18,FINJ8=19,FINJ9=20,FINJ10=21,FINJ11=22,FINJ12=23  sequence_type=Standard (Injector per cylinder)  behavior=Standard  update_mode=OS  granularity=Fine  use_makeup=off  min_eoi_soi_angle=90  use_diag=off  show_trans_enable=off  min_duration_mode=Static  min_duration=1.5  use_vardec=off  nam='INJ_'  read_level=1  write_level=1  group='System | I/O Pins | Injector Config'
  Spark Sequence : MotoHawk_lib/Advanced Digital I//O/Spark Sequence  text_resource=EST 1  code_resource=NONE  val_resource=-1  target=ECU565-128  resource_enum_str=(None)=-1,EST 1=36,EST 2=37,EST 3=38,EST 4=39,EST 5=40,EST 6=41,EST 7=42,EST 8=43,EST 9=44,EST 10=45,EST 11=46,EST 12=47,EST 13=48,EST 14=49,EST 15=50,EST 16=51  sequence_type=Standard (Coil per cylinder)  stop_mode=Angle Controlled  update_mode=OS  granularity=Fine  min_duration_mode=Static  min_duration=1.5  use_diag=off  open_threshold=500  use_vardec=off  nam='EST_'  read_level=1  write_level=1  group='System | I/O Pins | Spark Config'
  motohawk_TitleBlock : motohawk_annotations_lib/motohawk_TitleBlock  BlockType_='Mototron_Title_Block'  ttl=[get_param(bdroot, 'Description') '\rm\newlineSample H/W sensors, such as:\newlineA/D converters, digital inputs, frequency inputs, and engine encoder\newline']  copyright="'THE INFORMATION CONTAINED IN THIS\\newlineDRAWING IS THE SOLE PROPERTY OF\\newlineWOODWARD.  ANY REPRODUCTION IN\\newline PART OR AS A WHOLE WITHOUT THE\\newlineWRITTEN PERMISSION OF WOODWARD\\newline IS PROHIBITED.\\fontsize{16}\\rm\\copyright\\rm\\fontsize{10} 2009'"  address='\fontsize{22}\it\fontname{Arial Black}Woodward \fontname{Arial}\fontsize{10}\newline1000 East Drake Road, Fort Collins, CO, 80525\newlinemcs.woodward.com (866) 588-0494'  image_file='mh.jpg'  pretty_print=on  edit_text=|  edit_as=6
      | [get_param(bdroot, 'Description') '\rm
      | 
      | 
      | Sample H/W sensors, such as:
      | 
      | 
      | A/D converters, digital inputs, frequency inputs, and engine encoder
      | 
      | 
      | ']
  motohawk_calibration : MotoHawk_lib/Calibration & Probing Blocks/motohawk_calibration  nam='InjectorEnable'  val=false  storage=Display  show_more=on  name_source=Use Parameter  data_type=Inherit from 'Default Value'  read_level=1  write_level=1  ovr_cals=on  view_as=Enumeration  enum_struct={'Disabled', 'Enabled'}  vector_style=Wide Row  use_help_units=off  help=''  units=''  use_header_enum=off  row_header_enum={}  col_header_enum={}  use_min_max=off  min_val=-inf  max_val=inf  use_precision=off  precision=''  gain=1  offset=0  exp=1  use_mototune_group=off  mototune_group=motohawk_vardec_path(gcb)  data_stores=motohawk_sfun_calibration_data_stores
  motohawk_calibration1 : MotoHawk_lib/Calibration & Probing Blocks/motohawk_calibration  nam='SparkEnable'  val=false  storage=Display  show_more=on  name_source=Use Parameter  data_type=Inherit from 'Default Value'  read_level=1  write_level=1  ovr_cals=on  view_as=Enumeration  enum_struct={'Disabled', 'Enabled'}  vector_style=Wide Row  use_help_units=off  help=''  units=''  use_header_enum=off  row_header_enum={}  col_header_enum={}  use_min_max=off  min_val=-inf  max_val=inf  use_precision=off  precision=''  gain=1  offset=0  exp=1  use_mototune_group=off  mototune_group=motohawk_vardec_path(gcb)  data_stores=motohawk_sfun_calibration_data_stores
  motohawk_calibration2 : MotoHawk_lib/Calibration & Probing Blocks/motohawk_calibration  nam='SparkMaxDuration'  val=5000  storage=Calibration  show_more=on  name_source=Use Parameter  data_type=Inherit via back propagation  read_level=1  write_level=1  ovr_cals=on  view_as=Number  enum_struct={'Disabled', 'Enabled'}  vector_style=Wide Row  use_help_units=on  help="'Maximum duration for a spark pulse.  Must be a multiple of 5ms'"  units='us'  use_header_enum=off  row_header_enum={}  col_header_enum={}  use_min_max=off  min_val=-inf  max_val=inf  use_precision=off  precision=''  gain=1  offset=0  exp=1  use_mototune_group=off  mototune_group=motohawk_vardec_path(gcb)  data_stores=motohawk_sfun_calibration_data_stores
  motohawk_calibration3 : MotoHawk_lib/Calibration & Probing Blocks/motohawk_calibration  nam='InjectorMaxDuration'  val=500000  storage=Calibration  show_more=on  name_source=Use Parameter  data_type=Inherit via back propagation  read_level=1  write_level=1  ovr_cals=on  view_as=Number  enum_struct={'Disabled', 'Enabled'}  vector_style=Wide Row  use_help_units=on  help="'Maximum duration for an injector pulse.  Must be a multiple of 5ms'"  units='us'  use_header_enum=off  row_header_enum={}  col_header_enum={}  use_min_max=off  min_val=-inf  max_val=inf  use_precision=off  precision=''  gain=1  offset=0  exp=1  use_mototune_group=off  mototune_group=motohawk_vardec_path(gcb)  data_stores=motohawk_sfun_calibration_data_stores
  motohawk_calibration4 : MotoHawk_lib/Calibration & Probing Blocks/motohawk_calibration  nam='InjectorElectricalOffset'  val=0  storage=Calibration  show_more=on  name_source=Use Parameter  data_type=Inherit via back propagation  read_level=1  write_level=1  ovr_cals=on  view_as=Number  enum_struct={'Disabled', 'Enabled'}  vector_style=Wide Row  use_help_units=on  help='Extra duration added to each generated pulse to account for the injector turn on and turn off time'  units='us'  use_header_enum=off  row_header_enum={}  col_header_enum={}  use_min_max=off  min_val=-inf  max_val=inf  use_precision=off  precision=''  gain=1  offset=0  exp=1  use_mototune_group=off  mototune_group=motohawk_vardec_path(gcb)  data_stores=motohawk_sfun_calibration_data_stores
  motohawk_calibration5 : MotoHawk_lib/Calibration & Probing Blocks/motohawk_calibration  nam='InjectorPeakDuration'  val=0  storage=Calibration  show_more=on  name_source=Use Parameter  data_type=Inherit via back propagation  read_level=1  write_level=1  ovr_cals=on  view_as=Number  enum_struct={'Disabled', 'Enabled'}  vector_style=Wide Row  use_help_units=on  help='For a low-impedance injector using the peak-and-hold driver, the duration of the peak portion of the total injector pulse'  units='us'  use_header_enum=off  row_header_enum={}  col_header_enum={}  use_min_max=off  min_val=-inf  max_val=inf  use_precision=off  precision=''  gain=1  offset=0  exp=1  use_mototune_group=off  mototune_group=motohawk_vardec_path(gcb)  data_stores=motohawk_sfun_calibration_data_stores
  motohawk_callout1 : motohawk_annotations_lib/motohawk_callout1  BlockType_='Mototron_harea'  desc='Read from Bus of Actuators'  edit_text=Read from Bus of Actuators  edit_as=0
  motohawk_callout2 : motohawk_annotations_lib/motohawk_callout1  BlockType_='Mototron_harea'  desc='Convert from Engineering Units'  edit_text=Convert from Engineering Units  edit_as=0
  motohawk_callout3 : motohawk_annotations_lib/motohawk_callout1  BlockType_='Mototron_harea'  desc='Drive H/W Actuators'  edit_text=Drive H/W Actuators  edit_as=0
  motohawk_todo : motohawk_annotations_lib/motohawk_todo  BlockType_='Mototron_ToDo'  desc='\fontsize{16}\bfTo Do:\newlineAdd actuator blocks and\newlineconvert from engineering units'  edit_text=|  edit_as=2
      | \fontsize{16}\bfTo Do:
      | 
      | 
      | Add actuator blocks and
      | 
      | 
      | convert from engineering units
  wires:
  Actuators/1 -> Bus Selector/1
  Bus Selector/1 -> Gain/1  "<SparkStartAngle>"
  Bus Selector/2 -> Gain1/1  "<SparkStopAngle>"
  Gain/1 -> Data Type Conversion/1
  Gain1/1 -> Data Type Conversion1/1
  motohawk_calibration1/1 -> Spark Sequence/1
  Data Type Conversion/1 -> Spark Sequence/2
  Data Type Conversion1/1 -> Spark Sequence/3
  motohawk_calibration2/1 -> Spark Sequence/4
  Gain3/1 -> Data Type Conversion3/1
  Gain2/1 -> Data Type Conversion2/1
  Bus Selector/3 -> Gain2/1  "<FuelStartAngle>"
  Bus Selector/4 -> Gain3/1  "<FuelStopDuration>"
  Data Type Conversion2/1 -> Injector Sequence/2
  Data Type Conversion3/1 -> Injector Sequence/3
  motohawk_calibration3/1 -> Injector Sequence/5
  motohawk_calibration4/1 -> Injector Sequence/6
  motohawk_calibration5/1 -> Injector Sequence/4
  motohawk_calibration/1 -> Injector Sequence/1

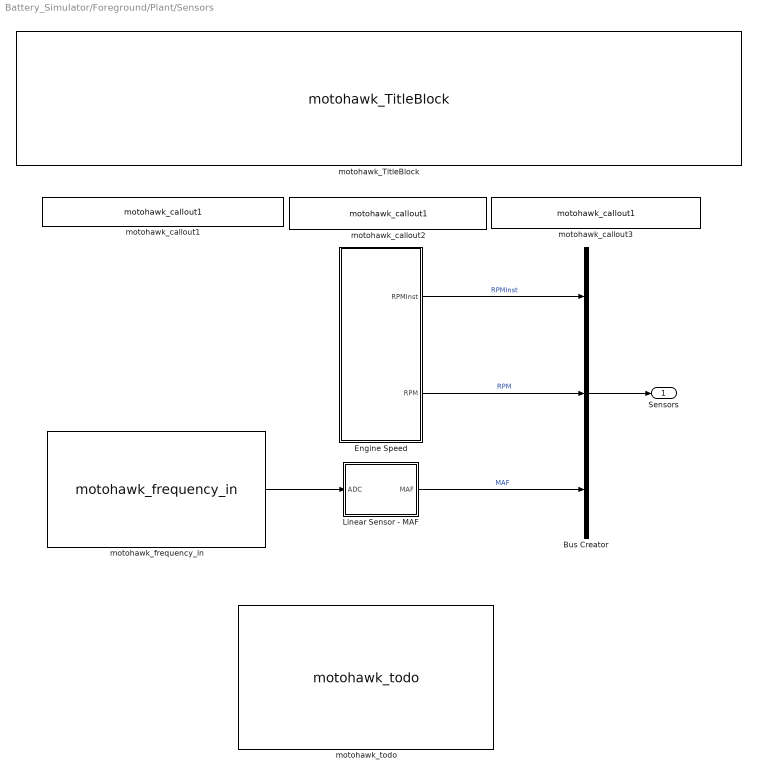
== system Battery_Simulator/Foreground/Plant/Sensors ==
  Bus Creator : BusCreator  Inputs=3
  Engine Speed : Subsystem
  Linear Sensor - MAF : Subsystem
  motohawk_TitleBlock : motohawk_annotations_lib/motohawk_TitleBlock  BlockType_='Mototron_Title_Block'  ttl=[get_param(bdroot, 'Description') '\rm\newlineSample H/W sensors, such as:\newlineA/D converters, digital inputs, frequency inputs, and engine encoder\newline']  copyright="'THE INFORMATION CONTAINED IN THIS\\newlineDRAWING IS THE SOLE PROPERTY OF\\newlineWOODWARD.  ANY REPRODUCTION IN\\newline PART OR AS A WHOLE WITHOUT THE\\newlineWRITTEN PERMISSION OF WOODWARD\\newline IS PROHIBITED.\\fontsize{16}\\rm\\copyright\\rm\\fontsize{10} 2009'"  address='\fontsize{22}\it\fontname{Arial Black}Woodward \fontname{Arial}\fontsize{10}\newline1000 East Drake Road, Fort Collins, CO, 80525\newlinemcs.woodward.com (866) 588-0494'  image_file='mh.jpg'  pretty_print=on  edit_text=|  edit_as=6
      | [get_param(bdroot, 'Description') '\rm
      | 
      | 
      | Sample H/W sensors, such as:
      | 
      | 
      | A/D converters, digital inputs, frequency inputs, and engine encoder
      | 
      | 
      | ']
  motohawk_callout1 : motohawk_annotations_lib/motohawk_callout1  BlockType_='Mototron_harea'  desc='Read from H/W'  edit_text=Read from H/W  edit_as=0
  motohawk_callout2 : motohawk_annotations_lib/motohawk_callout1  BlockType_='Mototron_harea'  desc='Convert to Engineering Units'  edit_text=Convert to Engineering Units  edit_as=0
  motohawk_callout3 : motohawk_annotations_lib/motohawk_callout1  BlockType_='Mototron_harea'  desc='Create a Bus of Sensors'  edit_text=Create a Bus of Sensors  edit_as=0
  motohawk_frequency_in : MotoHawk_lib/Advanced Digital I//O/motohawk_frequency_in  res_name=[]  text_resource=DG1M  code_resource=NONE  val_resource=-1  target=ECU565-128  resource_enum_str=(None)=-1,DG1M=93,DG2M=94,DG3M=95,DG4M=96,DG5M=102,DG6M=103,DG7M=104,SPD1=105,SPD2=106,DG8M=111  ipwm=No Duty Cycle Measurement  itrig=off  Nmax=8  edge=Rising Edge  alias=Disabled  min_freq=10  sig=Digital Input  use_avg=off  avg_mode=Fixed Interval  fixed_avg_pulses=2  use_vardec=off  use_cal=off  nam='FREQIN'  read_level=1  write_level=1  group='System | I/O Pins | Inputs Config'  cal_group='System | I/O Pins | Frequency In Config'
  motohawk_todo : motohawk_annotations_lib/motohawk_todo  BlockType_='Mototron_ToDo'  desc='\fontsize{16}\bfTo Do:\newlineAdd sensor blocks and\newlineconvert to engineering units'  edit_text=|  edit_as=2
      | \fontsize{16}\bfTo Do:
      | 
      | 
      | Add sensor blocks and
      | 
      | 
      | convert to engineering units
  Sensors : Outport
  wires:
  Bus Creator/1 -> Sensors/1
  Linear Sensor - MAF/1(MAF) -> Bus Creator/3  "MAF"
  Engine Speed/1(RPMInst) -> Bus Creator/1  "RPMInst"
  Engine Speed/2(RPM) -> Bus Creator/2  "RPM"
  motohawk_frequency_in/1 -> Linear Sensor - MAF/1(ADC)

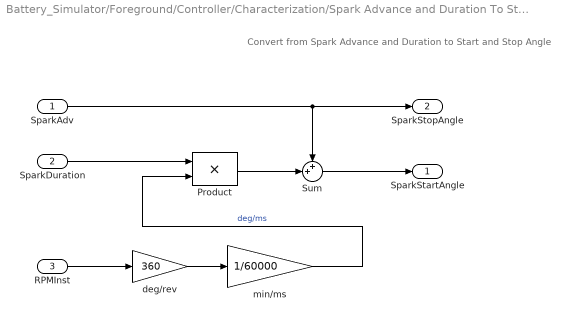
== system Battery_Simulator/Foreground/Controller/Characterization/Spark Advance and Duration To Start and Stop Angles ==
  note: Convert from Spark Advance and Duration
      | to Start and Stop Angle
  SparkAdv : Inport
  SparkDuration : Inport  Port=2
  RPMInst : Inport  Port=3
  Product : Product  InputSameDT=on  OutDataTypeStr=Inherit: Same as first input
  Sum : Sum  Inputs=++|  InputSameDT=on
  deg/rev : Gain  Gain=360  SaturateOnIntegerOverflow=on  OutDataTypeStr=Inherit: Same as input  ParamDataTypeStr=Inherit: Same as input
  min/ms : Gain  Gain=1/60000  SaturateOnIntegerOverflow=on  OutDataTypeStr=Inherit: Same as input  ParamDataTypeStr=Inherit: Same as input
  SparkStartAngle : Outport
  SparkStopAngle : Outport  Port=2
  wires:
  SparkAdv/1 -> SparkStopAngle/1, Sum/1
  RPMInst/1 -> deg/rev/1
  deg/rev/1 -> min/ms/1
  min/ms/1 -> Product/2  "deg/ms"
  SparkDuration/1 -> Product/1
  Sum/1 -> SparkStartAngle/1
  Product/1 -> Sum/2

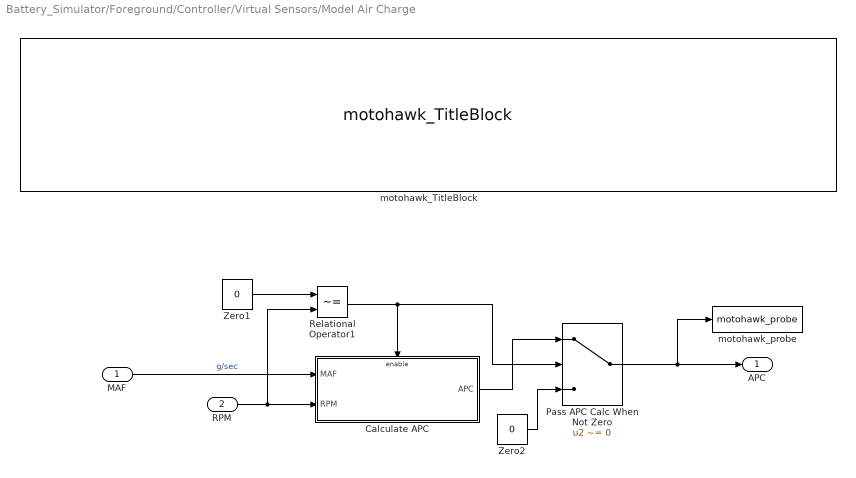
== system Battery_Simulator/Foreground/Controller/Virtual Sensors/Model Air Charge ==
  MAF : Inport
  RPM : Inport  Port=2
  Calculate APC : Subsystem
  Pass APC Calc When Not Zero : Switch  Criteria=u2 ~= 0  SaturateOnIntegerOverflow=on
  Relational Operator1 : RelationalOperator  Operator=~=
  Zero1 : Constant  Value=0  OutDataTypeStr=Inherit: Inherit via back propagation
  Zero2 : Constant  Value=0  OutDataTypeStr=Inherit: Inherit via back propagation
  motohawk_TitleBlock : motohawk_annotations_lib/motohawk_TitleBlock  BlockType_='Mototron_Title_Block'  ttl=[get_param(bdroot, 'Description') '\rm\newlineCompute Air Charge per Cylinder\newline(Grams / Event)\newline']  copyright="'THE INFORMATION CONTAINED IN THIS\\newlineDRAWING IS THE SOLE PROPERTY OF\\newlineWOODWARD.  ANY REPRODUCTION IN\\newline PART OR AS A WHOLE WITHOUT THE\\newlineWRITTEN PERMISSION OF WO0DWARD\\newline IS PROHIBITED.\\fontsize{16}\\rm\\copyright\\rm\\fontsize{10} 2009'"  address='\fontsize{22}\it\fontname{Arial Black}Woodward \fontname{Arial}\fontsize{10}\newline1000 East Drake Road, Fort Collins, CO, 80525\newlinemcs.woodward.com (866) 588-0494'  image_file='mh.jpg'  pretty_print=on  edit_text=|  edit_as=6
      | [get_param(bdroot, 'Description') '\rm
      | 
      | 
      | Compute Air Charge per Cylinder
      | 
      | 
      | (Grams / Event)
      | 
      | 
      | ']
  motohawk_probe : MotoHawk_lib/Calibration & Probing Blocks/motohawk_probe  nam='APC'  show_more=off  name_source=Use Parameter  read_level=1  view_as=Number  enum_struct={'Disabled', 'Enabled'}  vector_style=Wide Row  use_help_units=off  help=''  units=''  use_header_enum=off  row_header_enum={}  col_header_enum={}  use_min_max=off  min_val=-inf  max_val=inf  use_precision=off  precision=''  gain=1  offset=0  exp=1  use_mototune_group=off  mototune_group=motohawk_vardec_path(gcb)
  APC : Outport
  wires:
  MAF/1 -> Calculate APC/1(MAF)  "g/sec"
  RPM/1 -> Calculate APC/2(RPM), Relational Operator1/2
  Relational Operator1/1 -> Calculate APC/Enable, Pass APC Calc When Not Zero/2
  Zero1/1 -> Relational Operator1/1
  Pass APC Calc When Not Zero/1 -> APC/1, motohawk_probe/1
  Calculate APC/1(APC) -> Pass APC Calc When Not Zero/1
  Zero2/1 -> Pass APC Calc When Not Zero/3
